simulink model "sa1"  (R2022b)
settings: Solver=VariableStepAuto  StartTime=0.0  StopTime=25  RelTol=1e-3
settings Model: SimulationMode=accelerator  Creator=doshi  LastModifiedBy=doshi

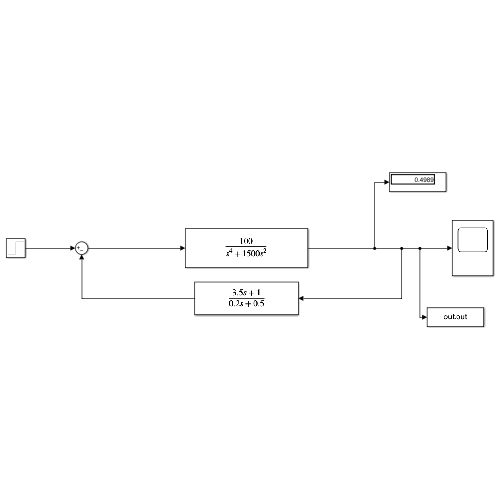
[thumbnail: Simulink's stored preview of the top-level diagram]
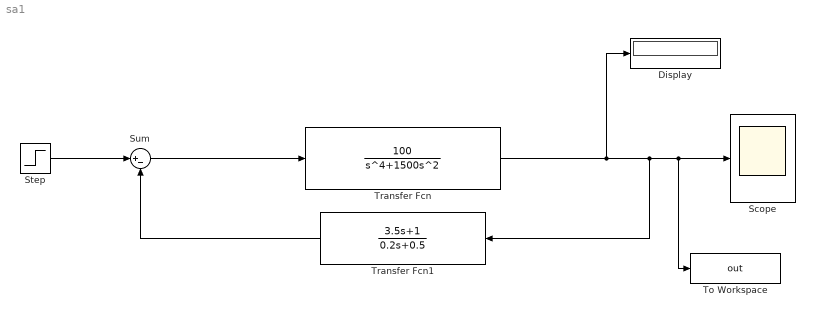
== system sa1 ==
  Display : Display
  Scope : Scope
  Step : Step  SampleTime=0
  Sum : Sum  Inputs=|+-
  To Workspace : ToWorkspace  VariableName=out  SaveFormat=Timeseries  SampleTime=-1
  Transfer Fcn : TransferFcn  Numerator=[100]  Denominator=[1 0 1500 0 0]
  Transfer Fcn1 : TransferFcn  Numerator=[3.5 1]  Denominator=[0.2 0.5]  ParameterTunability=Optimized
  wires:
  Transfer Fcn/1 -> Transfer Fcn1/1, To Workspace/1, Scope/1, Display/1
  Step/1 -> Sum/1
  Sum/1 -> Transfer Fcn/1
  Transfer Fcn1/1 -> Sum/2
